simulink library "vco_snn"  (R2023b)
settings: Solver=VariableStepAuto  StartTime=0.0  StopTime=10.0  RelTol=1e-3
libraries: simulink_extras x166, spsSeriesRLCBranchLib x132, spsControlledVoltageSourceLib x126, $bdroot x33, fl_lib x18, msbPllFoundation x10, nesl_utility x9, spsVoltageMeasurementLib x8, simulink x6, spsGroundLib x5, eeGeneralControl x2
(part 2 of 2)

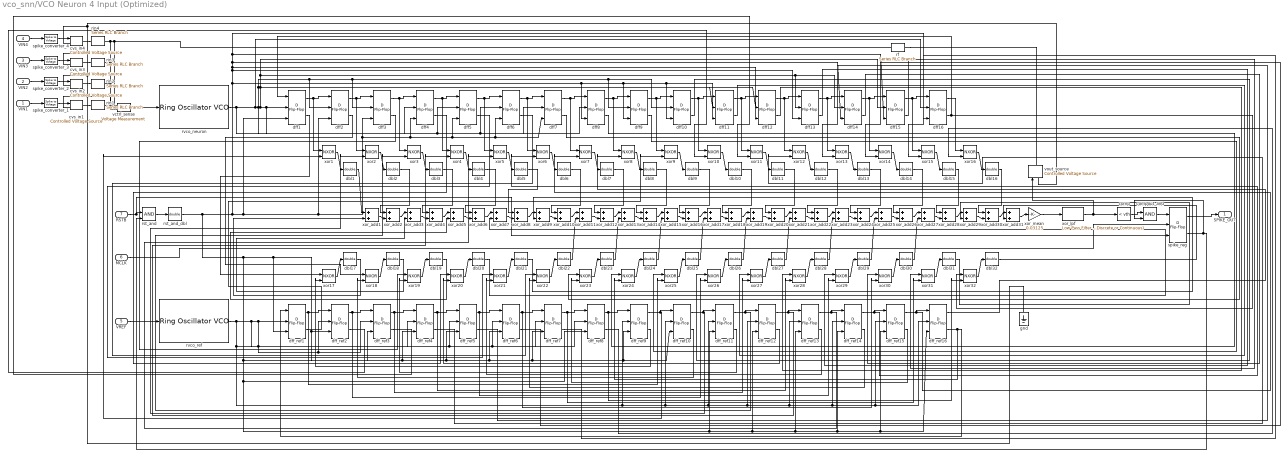
== system vco_snn/VCO Neuron 4 Input (Optimized) ==
  VIN1 : Inport
  VIN2 : Inport  Port=2
  VIN3 : Inport  Port=3
  VIN4 : Inport  Port=4
  VREF : Inport  Port=5
  MCLK : Inport  Port=6
  RSTB : Inport  Port=7
  comp : simulink/Logic and Bit Operations/Compare To Constant  relop=<  const=vth  OutDataTypeStr=boolean
  compout_and : Logic  IconShape=distinctive  AllPortsSameDT=off  OutDataTypeStr=boolean
  cvs_in{1..4} (4 alike) : spsControlledVoltageSourceLib/Controlled Voltage Source  Initialize=on  Source_Type=AC  Amplitude=0  Phase=0  Frequency=0  Measurements=None
  dbl{1..32} (32 alike) : DataTypeConversion  OutDataTypeStr=double  SaturateOnIntegerOverflow=off  RndMeth=Floor
  dff{1..16} (16 alike) : simulink_extras/Flip Flops/D Flip-Flop
  dff_ref{1..16} (16 alike) : simulink_extras/Flip Flops/D Flip-Flop
  gnd : spsGroundLib/Ground  LConnTagsString=a
  rf : spsSeriesRLCBranchLib/Series RLC Branch  LConnTagsString=__new0  RConnTagsString=__new0  BranchType=R  Resistance=rf  Inductance=1e-3  SetiL0=off  InitialCurrent=0  Capacitance=1e-6  Setx0=off  InitialVoltage=0  Measurements=None
  rin1 : spsSeriesRLCBranchLib/Series RLC Branch  LConnTagsString=__new0  RConnTagsString=__new0  BranchType=R  Resistance=rin1  Inductance=1e-3  SetiL0=off  InitialCurrent=0  Capacitance=1e-6  Setx0=off  InitialVoltage=0  Measurements=None
  rin2 : spsSeriesRLCBranchLib/Series RLC Branch  LConnTagsString=__new0  RConnTagsString=__new0  BranchType=R  Resistance=rin2  Inductance=1e-3  SetiL0=off  InitialCurrent=0  Capacitance=1e-6  Setx0=off  InitialVoltage=0  Measurements=None
  rin3 : spsSeriesRLCBranchLib/Series RLC Branch  LConnTagsString=__new0  RConnTagsString=__new0  BranchType=R  Resistance=rin3  Inductance=1e-3  SetiL0=off  InitialCurrent=0  Capacitance=1e-6  Setx0=off  InitialVoltage=0  Measurements=None
  rin4 : spsSeriesRLCBranchLib/Series RLC Branch  LConnTagsString=__new0  RConnTagsString=__new0  BranchType=R  Resistance=rin4  Inductance=1e-3  SetiL0=off  InitialCurrent=0  Capacitance=1e-6  Setx0=off  InitialVoltage=0  Measurements=None
  rst_and : Logic  IconShape=distinctive  AllPortsSameDT=off  OutDataTypeStr=boolean
  rst_and_dbl : DataTypeConversion  OutDataTypeStr=double  SaturateOnIntegerOverflow=off  RndMeth=Floor
  rvco_neuron : msbPllFoundation/Ring Oscillator VCO  SpecifyUsing=Voltage sensitivity  Kvco=kvco*32  Fo=(center_freq - (kvco/2))*32  ControlVoltage=[-5 0 5]  OutputFrequency=[2e9 2.5e9 3e9]  Amplitude=1  ExtraBuffer=off  NBuffer=10  AddPhaseNoise=off  SsbCheck=off  Foffset=[30e3 100e3 1e6 3e6 10e6]  PhaseNoise=[-56 -106 -132 -143 -152]  PeriodJitter=1.7e-15  CornerFrequency=5e5  CustomizeExponent=off  FlickerExponent=1.0  MaxKvco=320000000
  rvco_ref : msbPllFoundation/Ring Oscillator VCO  SpecifyUsing=Voltage sensitivity  Kvco=kvco*32  Fo=(center_freq - (kvco/2))*32  ControlVoltage=[-5 0 5]  OutputFrequency=[2e9 2.5e9 3e9]  Amplitude=1  ExtraBuffer=off  NBuffer=10  AddPhaseNoise=off  SsbCheck=off  Foffset=[30e3 100e3 1e6 3e6 10e6]  PhaseNoise=[-56 -106 -132 -143 -152]  PeriodJitter=1.7e-15  CornerFrequency=5e5  CustomizeExponent=off  FlickerExponent=1.0  MaxKvco=320000000
  spike_converter_1 : $bdroot/Spike to Voltage  vcm=vcm  spike_amp=spike_amp  sign=spike_sign1
  spike_converter_2 : $bdroot/Spike to Voltage  vcm=vcm  spike_amp=spike_amp  sign=spike_sign2
  spike_converter_3 : $bdroot/Spike to Voltage  vcm=vcm  spike_amp=spike_amp  sign=spike_sign3
  spike_converter_4 : $bdroot/Spike to Voltage  vcm=vcm  spike_amp=spike_amp  sign=spike_sign4
  spike_reg : simulink_extras/Flip Flops/D Flip-Flop
  vctrl_sense : spsVoltageMeasurementLib/Voltage Measurement  PhasorSimulation=off  OutputType=Complex  PSBequivalent=0
  vout_source : spsControlledVoltageSourceLib/Controlled Voltage Source  Initialize=on  Source_Type=AC  Amplitude=0  Phase=0  Frequency=0  Measurements=None
  xor{1..32} (32 alike) : Logic  Operator=NXOR  IconShape=distinctive  AllPortsSameDT=off  OutDataTypeStr=boolean
  xor_add{1..31} (31 alike) : Sum
  xor_lpf : eeGeneralControl/Low-Pass Filter (Discrete or Continuous)  K=1  T=xor_tau  B=inf  A=-inf  init_option=Inherited from block input  x0=0  Ts=0
  xor_mean : Gain  Gain=0.03125
  SPIKE_OUT : Outport
  wires:
  xor_add2/1 -> xor_add3/1
  dbl1/1 -> xor_add1/1
  xor17/1 -> dbl17/1
  dff_ref9/2 -> xor17/2
  spike_converter_2/1 -> cvs_in2/1
  xor8/1 -> dbl8/1
  dbl4/1 -> xor_add6/1
  xor_add5/1 -> xor_add6/2
  xor9/1 -> dbl9/1
  dff_ref13/2 -> xor21/2
  xor20/1 -> dbl20/1
  dff11/2 -> xor27/1
  dff10/2 -> xor26/1
  xor_add25/1 -> xor_add26/2
  dff4/2 -> xor20/1
  xor_add13/1 -> xor_add14/2
  dff_ref3/2 -> xor11/2
  spike_converter_3/1 -> cvs_in3/1
  dbl29/1 -> xor_add25/2
  xor18/1 -> dbl18/1
  xor_add4/1 -> xor_add5/1
  dbl9/1 -> xor_add16/1
  dff3/2 -> xor19/1
  dbl31/1 -> xor_add29/2
  dbl11/1 -> xor_add20/1
  spike_reg/2 -> compout_and/2, rst_and/2
  xor_add26/1 -> xor_add27/1
  dbl22/1 -> xor_add11/2
  xor_add15/1 -> xor_add16/2
  dff9/2 -> xor25/1
  dbl5/1 -> xor_add8/1
  xor7/1 -> dbl7/1
  xor3/1 -> dbl3/1
  xor5/1 -> dbl5/1
  xor_add7/1 -> xor_add8/2
  dff_ref11/2 -> xor19/2
  dff_ref8/2 -> xor16/2
  xor_add1/1 -> xor_add2/2
  spike_converter_4/1 -> cvs_in4/1
  dff_ref15/1 -> dff_ref16/1, xor7/2
  dff14/2 -> xor30/1
  xor_add12/1 -> xor_add13/1
  dbl23/1 -> xor_add13/2
  dff_ref5/2 -> xor13/2
  dbl13/1 -> xor_add24/1
  xor30/1 -> dbl30/1
  xor_add23/1 -> xor_add24/2
  xor22/1 -> dbl22/1
  xor12/1 -> dbl12/1
  xor15/1 -> dbl15/1
  dff_ref4/2 -> xor12/2
  dff_ref3/1 -> dff_ref4/1, xor27/2
  spike_reg/1 -> SPIKE_OUT/1
  xor24/1 -> dbl24/1
  xor_add9/1 -> xor_add10/2
  dff_ref12/1 -> dff_ref13/1, xor4/2
  xor28/1 -> dbl28/1
  xor_add19/1 -> xor_add20/2
  VIN1/1 -> spike_converter_1/1
  xor_add20/1 -> xor_add21/1
  xor_add11/1 -> xor_add12/2
  dff16/1 -> xor16/1
  dff6/1 -> dff7/1, xor6/1
  dff3/1 -> dff4/1, xor3/1
  dbl18/1 -> xor_add3/2
  xor27/1 -> dbl27/1
  xor_lpf/1 -> vout_source/1, comp/1
  dbl28/1 -> xor_add23/2
  dff_ref14/2 -> xor22/2
  dff1/1 -> dff2/1, xor1/1
  dbl3/1 -> xor_add4/1
  xor32/1 -> dbl32/1
  dff_ref15/2 -> xor23/2
  xor_add8/1 -> xor_add9/1
  xor_add6/1 -> xor_add7/1
  xor14/1 -> dbl14/1
  dff_ref11/1 -> dff_ref12/1, xor3/2
  xor1/1 -> dbl1/1
  dff6/2 -> xor22/1
  xor_add10/1 -> xor_add11/1
  dbl27/1 -> xor_add21/2
  xor16/1 -> dbl16/1
  xor29/1 -> dbl29/1
  dff15/1 -> dff16/1, xor15/1
  dff5/2 -> xor21/1
  dbl14/1 -> xor_add26/1
  xor_add21/1 -> xor_add22/2
  dbl17/1 -> xor_add1/2
  dff7/2 -> xor23/1
  dff_ref7/2 -> xor15/2
  dff14/1 -> dff15/1, xor14/1
  dff_ref16/1 -> xor8/2
  dff_ref1/1 -> dff_ref2/1, xor25/2
  dff_ref1/2 -> xor9/2
  rst_and/1 -> rst_and_dbl/1
  dbl19/1 -> xor_add5/2
  dbl6/1 -> xor_add10/1
  VIN2/1 -> spike_converter_2/1
  dff_ref9/1 -> dff_ref10/1, xor1/2
  dff_ref14/1 -> dff_ref15/1, xor6/2
  xor10/1 -> dbl10/1
  xor_mean/1 -> xor_lpf/1
  xor_add27/1 -> xor_add28/2
  dff_ref10/2 -> xor18/2
  xor2/1 -> dbl2/1
  dff16/2 -> dff1/1, xor32/1
  dbl20/1 -> xor_add7/2
  xor13/1 -> dbl13/1
  dbl16/1 -> xor_add30/1
  dff2/1 -> dff3/1, xor2/1
  dff10/1 -> dff11/1, xor10/1
  rst_and_dbl/1 -> dff_ref15/3, dff_ref16/3, dff_ref14/3, dff_ref13/3, dff_ref12/3, dff_ref11/3, dff_ref8/3, dff_ref9/3, dff_ref10/3, dff_ref7/3, dff_ref6/3, dff_ref5/3, dff_ref4/3, dff_ref2/3, dff_ref3/3, dff_ref1/3, dff6/3, dff7/3, dff5/3, dff4/3, dff3/3, dff2/3, dff1/3, dff10/3, dff11/3, dff9/3, dff8/3, dff15/3, dff16/3, dff14/3, dff12/3, dff13/3
  xor_add22/1 -> xor_add23/1
  dff_ref12/2 -> xor20/2
  RSTB/1 -> rst_and/1, spike_reg/3
  dff8/1 -> dff9/1, xor8/1
  dff_ref6/2 -> xor14/2
  xor_add31/1 -> xor_mean/1
  xor_add24/1 -> xor_add25/1
  xor_add30/1 -> xor_add31/1
  dbl25/1 -> xor_add17/2
  comp/1 -> compout_and/1
  dff_ref13/1 -> dff_ref14/1, xor5/2
  dff_ref8/1 -> dff_ref9/1, xor32/2
  xor_add29/1 -> xor_add30/2
  xor_add28/1 -> xor_add29/1
  dbl8/1 -> xor_add14/1
  dff_ref4/1 -> dff_ref5/1, xor28/2
  dff_ref10/1 -> dff_ref11/1, xor2/2
  VIN4/1 -> spike_converter_4/1
  xor31/1 -> dbl31/1
  dff11/1 -> dff12/1, xor11/1
  dff1/2 -> xor17/1
  xor11/1 -> dbl11/1
  dbl32/1 -> xor_add31/2
  dff12/1 -> dff13/1, xor12/1
  VIN3/1 -> spike_converter_3/1
  dff_ref16/2 -> dff_ref1/1, xor24/2
  dff7/1 -> dff8/1, xor7/1
  xor_add14/1 -> xor_add15/1
  spike_converter_1/1 -> cvs_in1/1
  dbl21/1 -> xor_add9/2
  dbl12/1 -> xor_add22/1
  xor25/1 -> dbl25/1
  dff4/1 -> dff5/1, xor4/1
  xor_add16/1 -> xor_add17/1
  xor_add17/1 -> xor_add18/2
  dff5/1 -> dff6/1, xor5/1
  dff8/2 -> xor24/1
  xor_add18/1 -> xor_add19/1
  rvco_neuron/1 -> dff6/2, dff7/2, dff5/2, dff1/2, dff8/2, dff13/2, dff14/2, dff15/2, dff12/2, dff9/2, dff10/2, dff3/2, dff2/2, dff11/2, dff4/2, dff16/2
  xor4/1 -> dbl4/1
  dff15/2 -> xor31/1
  xor19/1 -> dbl19/1
  dff13/2 -> xor29/1
  dff_ref6/1 -> dff_ref7/1, xor30/2
  dbl30/1 -> xor_add27/2
  dbl15/1 -> xor_add28/1
  dff_ref2/2 -> xor10/2
  dbl7/1 -> xor_add12/1
  dbl2/1 -> xor_add2/1
  dbl10/1 -> xor_add18/1
  dff13/1 -> dff14/1, xor13/1
  dff_ref2/1 -> dff_ref3/1, xor26/2
  dff12/2 -> xor28/1
  compout_and/1 -> spike_reg/1
  dff9/1 -> dff10/1, xor9/1
  xor_add3/1 -> xor_add4/2
  vctrl_sense/1 -> rvco_neuron/1
  dbl24/1 -> xor_add15/2
  rvco_ref/1 -> dff_ref15/2, dff_ref16/2, dff_ref14/2, dff_ref13/2, dff_ref12/2, dff_ref11/2, dff_ref10/2, dff_ref9/2, dff_ref8/2, dff_ref6/2, dff_ref7/2, dff_ref5/2, dff_ref2/2, dff_ref3/2, dff_ref4/2, dff_ref1/2
  dff_ref7/1 -> dff_ref8/1, xor31/2
  dff2/2 -> xor18/1
  dff_ref5/1 -> dff_ref6/1, xor29/2
  xor21/1 -> dbl21/1
  dbl26/1 -> xor_add19/2
  MCLK/1 -> spike_reg/2
  VREF/1 -> rvco_ref/1
  xor6/1 -> dbl6/1
  xor26/1 -> dbl26/1
  xor23/1 -> dbl23/1
  connections:
  cvs_in2/RConn1 -- rin2/LConn1
  rf/LConn1 -- rin1/RConn1 -- rin4/RConn1 -- rin3/RConn1 -- rin2/RConn1 -- vctrl_sense/LConn1
  cvs_in4/RConn1 -- rin4/LConn1
  rf/RConn1 -- vout_source/RConn1
  cvs_in3/RConn1 -- rin3/LConn1
  cvs_in1/RConn1 -- rin1/LConn1
  cvs_in1/LConn1 -- vctrl_sense/LConn2 -- gnd/LConn1 -- cvs_in2/LConn1 -- cvs_in3/LConn1 -- cvs_in4/LConn1 -- vout_source/LConn1

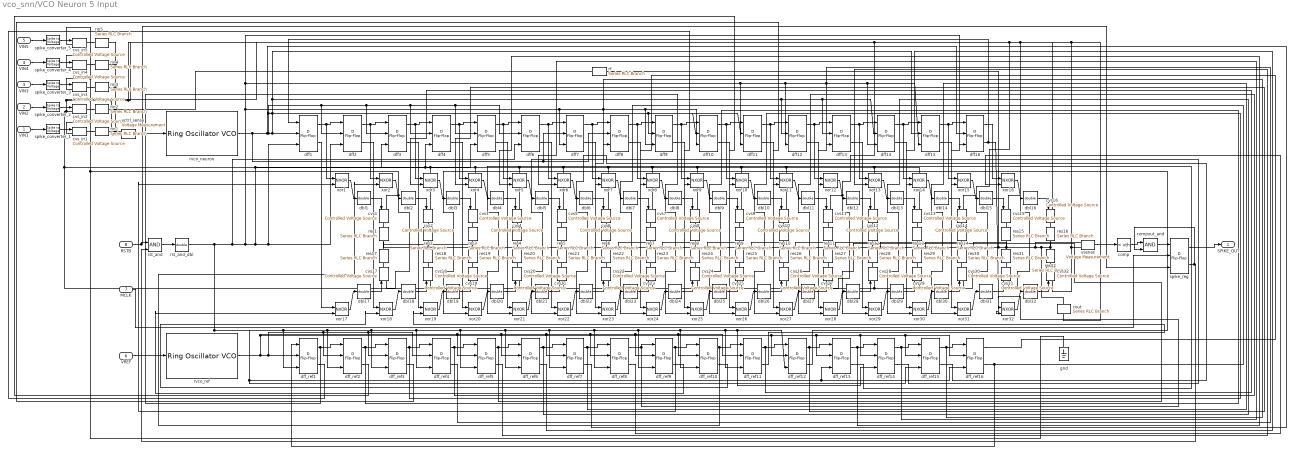
== system vco_snn/VCO Neuron 5 Input ==
  VIN1 : Inport
  VIN2 : Inport  Port=2
  VIN3 : Inport  Port=3
  VIN4 : Inport  Port=4
  VIN5 : Inport  Port=5
  VREF : Inport  Port=6
  MCLK : Inport  Port=7
  RSTB : Inport  Port=8
  comp : simulink/Logic and Bit Operations/Compare To Constant  relop=<  const=vth  OutDataTypeStr=boolean
  compout_and : Logic  IconShape=distinctive  AllPortsSameDT=off  OutDataTypeStr=boolean
  cout : spsSeriesRLCBranchLib/Series RLC Branch  LConnTagsString=__new0  RConnTagsString=__new0  BranchType=C  Resistance=1  Inductance=1e-3  SetiL0=off  InitialCurrent=0  Capacitance=vout_cap  Setx0=on  InitialVoltage=0.5  Measurements=None
  cvs{1..32} (32 alike) : spsControlledVoltageSourceLib/Controlled Voltage Source  Initialize=on  Source_Type=AC  Amplitude=0  Phase=0  Frequency=0  Measurements=None
  cvs_in{1..5} (5 alike) : spsControlledVoltageSourceLib/Controlled Voltage Source  Initialize=on  Source_Type=AC  Amplitude=0  Phase=0  Frequency=0  Measurements=None
  dbl{1..32} (32 alike) : DataTypeConversion  OutDataTypeStr=double  SaturateOnIntegerOverflow=off  RndMeth=Floor
  dff{1..16} (16 alike) : simulink_extras/Flip Flops/D Flip-Flop
  dff_ref{1..16} (16 alike) : simulink_extras/Flip Flops/D Flip-Flop
  gnd : spsGroundLib/Ground  LConnTagsString=a
  res{1..32} (32 alike) : spsSeriesRLCBranchLib/Series RLC Branch  LConnTagsString=__new0  RConnTagsString=__new0  BranchType=R  Resistance=xor_res  Inductance=1e-3  SetiL0=off  InitialCurrent=0  Capacitance=1e-6  Setx0=off  InitialVoltage=0  Measurements=None
  rf : spsSeriesRLCBranchLib/Series RLC Branch  LConnTagsString=__new0  RConnTagsString=__new0  BranchType=R  Resistance=rf  Inductance=1e-3  SetiL0=off  InitialCurrent=0  Capacitance=1e-6  Setx0=off  InitialVoltage=0  Measurements=None
  rin1 : spsSeriesRLCBranchLib/Series RLC Branch  LConnTagsString=__new0  RConnTagsString=__new0  BranchType=R  Resistance=rin1  Inductance=1e-3  SetiL0=off  InitialCurrent=0  Capacitance=1e-6  Setx0=off  InitialVoltage=0  Measurements=None
  rin2 : spsSeriesRLCBranchLib/Series RLC Branch  LConnTagsString=__new0  RConnTagsString=__new0  BranchType=R  Resistance=rin2  Inductance=1e-3  SetiL0=off  InitialCurrent=0  Capacitance=1e-6  Setx0=off  InitialVoltage=0  Measurements=None
  rin3 : spsSeriesRLCBranchLib/Series RLC Branch  LConnTagsString=__new0  RConnTagsString=__new0  BranchType=R  Resistance=rin3  Inductance=1e-3  SetiL0=off  InitialCurrent=0  Capacitance=1e-6  Setx0=off  InitialVoltage=0  Measurements=None
  rin4 : spsSeriesRLCBranchLib/Series RLC Branch  LConnTagsString=__new0  RConnTagsString=__new0  BranchType=R  Resistance=rin4  Inductance=1e-3  SetiL0=off  InitialCurrent=0  Capacitance=1e-6  Setx0=off  InitialVoltage=0  Measurements=None
  rin5 : spsSeriesRLCBranchLib/Series RLC Branch  LConnTagsString=__new0  RConnTagsString=__new0  BranchType=R  Resistance=rin5  Inductance=1e-3  SetiL0=off  InitialCurrent=0  Capacitance=1e-6  Setx0=off  InitialVoltage=0  Measurements=None
  rst_and : Logic  IconShape=distinctive  AllPortsSameDT=off  OutDataTypeStr=boolean
  rst_and_dbl : DataTypeConversion  OutDataTypeStr=double  SaturateOnIntegerOverflow=off  RndMeth=Floor
  rvco_neuron : msbPllFoundation/Ring Oscillator VCO  SpecifyUsing=Voltage sensitivity  Kvco=kvco*32  Fo=(center_freq - (kvco/2))*32  ControlVoltage=[-5 0 5]  OutputFrequency=[2e9 2.5e9 3e9]  Amplitude=1  ExtraBuffer=off  NBuffer=10  AddPhaseNoise=off  SsbCheck=off  Foffset=[30e3 100e3 1e6 3e6 10e6]  PhaseNoise=[-56 -106 -132 -143 -152]  PeriodJitter=1.7e-15  CornerFrequency=5e5  CustomizeExponent=off  FlickerExponent=1.0  MaxKvco=320000000
  rvco_ref : msbPllFoundation/Ring Oscillator VCO  SpecifyUsing=Voltage sensitivity  Kvco=kvco*32  Fo=(center_freq - (kvco/2))*32  ControlVoltage=[-5 0 5]  OutputFrequency=[2e9 2.5e9 3e9]  Amplitude=1  ExtraBuffer=off  NBuffer=10  AddPhaseNoise=off  SsbCheck=off  Foffset=[30e3 100e3 1e6 3e6 10e6]  PhaseNoise=[-56 -106 -132 -143 -152]  PeriodJitter=1.7e-15  CornerFrequency=5e5  CustomizeExponent=off  FlickerExponent=1.0  MaxKvco=320000000
  spike_converter_1 : $bdroot/Spike to Voltage  vcm=vcm  spike_amp=spike_amp  sign=spike_sign1
  spike_converter_2 : $bdroot/Spike to Voltage  vcm=vcm  spike_amp=spike_amp  sign=spike_sign2
  spike_converter_3 : $bdroot/Spike to Voltage  vcm=vcm  spike_amp=spike_amp  sign=spike_sign3
  spike_converter_4 : $bdroot/Spike to Voltage  vcm=vcm  spike_amp=spike_amp  sign=spike_sign4
  spike_converter_5 : $bdroot/Spike to Voltage  vcm=vcm  spike_amp=spike_amp  sign=spike_sign5
  spike_reg : simulink_extras/Flip Flops/D Flip-Flop
  vctrl_sense : spsVoltageMeasurementLib/Voltage Measurement  PhasorSimulation=off  OutputType=Complex  PSBequivalent=0
  vsense : spsVoltageMeasurementLib/Voltage Measurement  PhasorSimulation=off  OutputType=Complex  PSBequivalent=0
  xor{1..32} (32 alike) : Logic  Operator=NXOR  IconShape=distinctive  AllPortsSameDT=off  OutDataTypeStr=boolean
  SPIKE_OUT : Outport
  wires:
  xor31/1 -> dbl31/1
  dbl17/1 -> cvs17/1
  xor8/1 -> dbl8/1
  xor18/1 -> dbl18/1
  dbl19/1 -> cvs19/1
  xor17/1 -> dbl17/1
  xor22/1 -> dbl22/1
  dbl21/1 -> cvs21/1
  dbl6/1 -> cvs6/1
  dff_ref15/2 -> xor23/2
  dbl7/1 -> cvs7/1
  dbl5/1 -> cvs5/1
  xor30/1 -> dbl30/1
  xor3/1 -> dbl3/1
  VREF/1 -> rvco_ref/1
  dff11/2 -> xor27/1
  dff2/1 -> dff3/1, xor2/1
  xor25/1 -> dbl25/1
  xor24/1 -> dbl24/1
  spike_reg/1 -> SPIKE_OUT/1
  dff_ref16/2 -> dff_ref1/1, xor24/2
  rst_and/1 -> rst_and_dbl/1
  dbl3/1 -> cvs3/1
  dff8/1 -> dff9/1, xor8/1
  dff_ref9/2 -> xor17/2
  dff4/2 -> xor20/1
  dbl15/1 -> cvs15/1
  dff8/2 -> xor24/1
  xor32/1 -> dbl32/1
  dbl18/1 -> cvs18/1
  dff_ref13/1 -> dff_ref14/1, xor5/2
  dff3/2 -> xor19/1
  dbl10/1 -> cvs10/1
  dbl26/1 -> cvs26/1
  dff_ref7/2 -> xor15/2
  dbl25/1 -> cvs25/1
  dbl24/1 -> cvs24/1
  xor12/1 -> dbl12/1
  xor28/1 -> dbl28/1
  VIN5/1 -> spike_converter_5/1
  dff12/2 -> xor28/1
  dbl22/1 -> cvs22/1
  compout_and/1 -> spike_reg/1
  dbl13/1 -> cvs13/1
  dff_ref7/1 -> dff_ref8/1, xor31/2
  dff3/1 -> dff4/1, xor3/1
  dff_ref15/1 -> dff_ref16/1, xor7/2
  xor19/1 -> dbl19/1
  dff14/2 -> xor30/1
  xor15/1 -> dbl15/1
  spike_converter_3/1 -> cvs_in3/1
  dff_ref9/1 -> dff_ref10/1, xor1/2
  dbl16/1 -> cvs16/1
  dff_ref3/1 -> dff_ref4/1, xor27/2
  dff13/1 -> dff14/1, xor13/1
  dff9/1 -> dff10/1, xor9/1
  xor14/1 -> dbl14/1
  dff1/1 -> dff2/1, xor1/1
  dff_ref2/1 -> dff_ref3/1, xor26/2
  dff5/1 -> dff6/1, xor5/1
  dff_ref5/1 -> dff_ref6/1, xor29/2
  dff_ref11/1 -> dff_ref12/1, xor3/2
  spike_reg/2 -> compout_and/2, rst_and/2
  dff6/1 -> dff7/1, xor6/1
  dff12/1 -> dff13/1, xor12/1
  dff_ref8/2 -> xor16/2
  spike_converter_5/1 -> cvs_in5/1
  dbl1/1 -> cvs1/1
  dff16/1 -> xor16/1
  dff_ref12/1 -> dff_ref13/1, xor4/2
  dff10/1 -> dff11/1, xor10/1
  dff10/2 -> xor26/1
  dff_ref1/1 -> dff_ref2/1, xor25/2
  xor20/1 -> dbl20/1
  dff14/1 -> dff15/1, xor14/1
  VIN3/1 -> spike_converter_3/1
  dff13/2 -> xor29/1
  dff_ref14/2 -> xor22/2
  dff_ref3/2 -> xor11/2
  spike_converter_2/1 -> cvs_in2/1
  VIN4/1 -> spike_converter_4/1
  xor27/1 -> dbl27/1
  vsense/1 -> comp/1
  spike_converter_4/1 -> cvs_in4/1
  RSTB/1 -> rst_and/1, spike_reg/3
  dff7/1 -> dff8/1, xor7/1
  xor7/1 -> dbl7/1
  dff_ref6/1 -> dff_ref7/1, xor30/2
  dff_ref14/1 -> dff_ref15/1, xor6/2
  comp/1 -> compout_and/1
  xor9/1 -> dbl9/1
  dff16/2 -> dff1/1, xor32/1
  dff_ref4/1 -> dff_ref5/1, xor28/2
  xor5/1 -> dbl5/1
  dbl32/1 -> cvs32/1
  xor13/1 -> dbl13/1
  dff_ref5/2 -> xor13/2
  xor11/1 -> dbl11/1
  dbl2/1 -> cvs2/1
  xor16/1 -> dbl16/1
  xor2/1 -> dbl2/1
  xor21/1 -> dbl21/1
  dff15/2 -> xor31/1
  vctrl_sense/1 -> rvco_neuron/1
  dbl8/1 -> cvs8/1
  dff1/2 -> xor17/1
  xor4/1 -> dbl4/1
  VIN1/1 -> spike_converter_1/1
  dff_ref1/2 -> xor9/2
  MCLK/1 -> spike_reg/2
  dff5/2 -> xor21/1
  dbl29/1 -> cvs29/1
  xor29/1 -> dbl29/1
  dff_ref12/2 -> xor20/2
  dff15/1 -> dff16/1, xor15/1
  dbl30/1 -> cvs30/1
  dff_ref11/2 -> xor19/2
  dbl9/1 -> cvs9/1
  xor6/1 -> dbl6/1
  spike_converter_1/1 -> cvs_in1/1
  dbl28/1 -> cvs28/1
  rst_and_dbl/1 -> dff_ref13/3, dff_ref16/3, dff_ref15/3, dff_ref12/3, dff_ref14/3, dff_ref11/3, dff_ref10/3, dff_ref9/3, dff_ref8/3, dff_ref7/3, dff_ref6/3, dff_ref5/3, dff_ref4/3, dff_ref3/3, dff_ref2/3, dff_ref1/3, dff1/3, dff2/3, dff4/3, dff5/3, dff3/3, dff9/3, dff10/3, dff8/3, dff7/3, dff14/3, dff15/3, dff13/3, dff12/3, dff11/3, dff16/3, dff6/3
  dff7/2 -> xor23/1
  xor10/1 -> dbl10/1
  rvco_ref/1 -> dff_ref3/2, dff_ref4/2, dff_ref2/2, dff_ref1/2, dff_ref15/2, dff_ref16/2, dff_ref14/2, dff_ref13/2, dff_ref12/2, dff_ref10/2, dff_ref11/2, dff_ref9/2, dff_ref8/2, dff_ref7/2, dff_ref6/2, dff_ref5/2
  VIN2/1 -> spike_converter_2/1
  xor26/1 -> dbl26/1
  dbl4/1 -> cvs4/1
  dff_ref2/2 -> xor10/2
  dff_ref16/1 -> xor8/2
  dbl11/1 -> cvs11/1
  dff_ref8/1 -> dff_ref9/1, xor32/2
  xor1/1 -> dbl1/1
  dbl31/1 -> cvs31/1
  dff_ref13/2 -> xor21/2
  dff6/2 -> xor22/1
  xor23/1 -> dbl23/1
  dbl20/1 -> cvs20/1
  dbl12/1 -> cvs12/1
  dbl23/1 -> cvs23/1
  dff11/1 -> dff12/1, xor11/1
  dff9/2 -> xor25/1
  dff_ref4/2 -> xor12/2
  dff_ref6/2 -> xor14/2
  dff4/1 -> dff5/1, xor4/1
  dbl14/1 -> cvs14/1
  rvco_neuron/1 -> dff7/2, dff8/2, dff13/2, dff14/2, dff12/2, dff15/2, dff11/2, dff1/2, dff9/2, dff10/2, dff5/2, dff6/2, dff4/2, dff3/2, dff2/2, dff16/2
  dff_ref10/2 -> xor18/2
  dbl27/1 -> cvs27/1
  dff2/2 -> xor18/1
  dff_ref10/1 -> dff_ref11/1, xor2/2
  connections:
  cvs21/RConn1 -- res21/RConn1
  cvs27/RConn1 -- res27/RConn1
  cvs18/RConn1 -- res18/RConn1
  cvs30/RConn1 -- res30/RConn1
  cvs2/RConn1 -- res2/RConn1
  cvs25/RConn1 -- res25/RConn1
  cvs15/RConn1 -- res15/RConn1
  cvs23/RConn1 -- res23/RConn1
  cvs8/RConn1 -- res8/RConn1
  cvs5/RConn1 -- res5/RConn1
  cvs16/RConn1 -- res16/RConn1
  cvs28/RConn1 -- res28/RConn1
  cvs_in4/RConn1 -- rin4/LConn1
  cvs14/RConn1 -- res14/RConn1
  cvs10/RConn1 -- res10/RConn1
  cvs31/RConn1 -- res31/RConn1
  cvs11/RConn1 -- res11/RConn1
  cvs_in1/RConn1 -- rin1/LConn1
  cvs3/RConn1 -- res3/RConn1
  cvs4/RConn1 -- res4/RConn1
  cvs9/RConn1 -- res9/RConn1
  rin1/RConn1 -- vctrl_sense/LConn1 -- rin2/RConn1 -- rf/LConn1 -- rin3/RConn1 -- rin5/RConn1 -- rin4/RConn1
  cvs7/RConn1 -- res7/RConn1
  cvs12/RConn1 -- res12/RConn1
  cvs32/RConn1 -- res32/RConn1
  cvs19/RConn1 -- res19/RConn1
  cvs26/RConn1 -- res26/RConn1
  cvs_in2/RConn1 -- rin2/LConn1
  cvs20/RConn1 -- res20/RConn1
  cvs13/RConn1 -- res13/RConn1
  cvs29/RConn1 -- res29/RConn1
  cvs24/RConn1 -- res24/RConn1
  cvs13/LConn1 -- cvs12/LConn1 -- cvs10/LConn1 -- cvs9/LConn1 -- cvs8/LConn1 -- cvs7/LConn1 -- cvs6/LConn1 -- cvs5/LConn1 -- cvs4/LConn1 -- cvs3/LConn1 -- cvs2/LConn1 -- cvs17/LConn1 -- cvs1/LConn1 -- gnd/LConn1 -- cvs_in1/LConn1 -- cvs27/LConn1 -- cvs11/LConn1 -- cvs15/LConn1 -- cvs14/LConn1 -- cvs32/LConn1 -- vsense/LConn2 -- cout/RConn1 -- cvs31/LConn1 -- cvs30/LConn1 -- vctrl_sense/LConn2 -- cvs_in5/LConn1 -- cvs_in4/LConn1 -- cvs_in3/LConn1 -- cvs16/LConn1 -- cvs_in2/LConn1 -- cvs18/LConn1 -- cvs19/LConn1 -- cvs20/LConn1 -- cvs21/LConn1 -- cvs22/LConn1 -- cvs23/LConn1 -- cvs24/LConn1 -- cvs25/LConn1 -- cvs26/LConn1 -- cvs29/LConn1 -- cvs28/LConn1
  cvs_in3/RConn1 -- rin3/LConn1
  cvs_in5/RConn1 -- rin5/LConn1
  cvs22/RConn1 -- res22/RConn1
  cvs17/RConn1 -- res17/RConn1
  cvs1/RConn1 -- res1/RConn1
  res2/LConn1 -- res1/LConn1 -- res18/LConn1 -- res17/LConn1 -- res19/LConn1 -- res3/LConn1 -- res20/LConn1 -- res4/LConn1 -- res21/LConn1 -- res5/LConn1 -- res22/LConn1 -- res6/LConn1 -- res23/LConn1 -- res7/LConn1 -- res24/LConn1 -- res8/LConn1 -- res25/LConn1 -- res9/LConn1 -- res26/LConn1 -- res10/LConn1 -- res27/LConn1 -- res11/LConn1 -- res28/LConn1 -- res12/LConn1 -- res29/LConn1 -- res13/LConn1 -- res30/LConn1 -- res14/LConn1 -- res31/LConn1 -- rf/RConn1 -- res15/LConn1 -- vsense/LConn1 -- cout/LConn1 -- res32/LConn1 -- res16/LConn1
  cvs6/RConn1 -- res6/RConn1

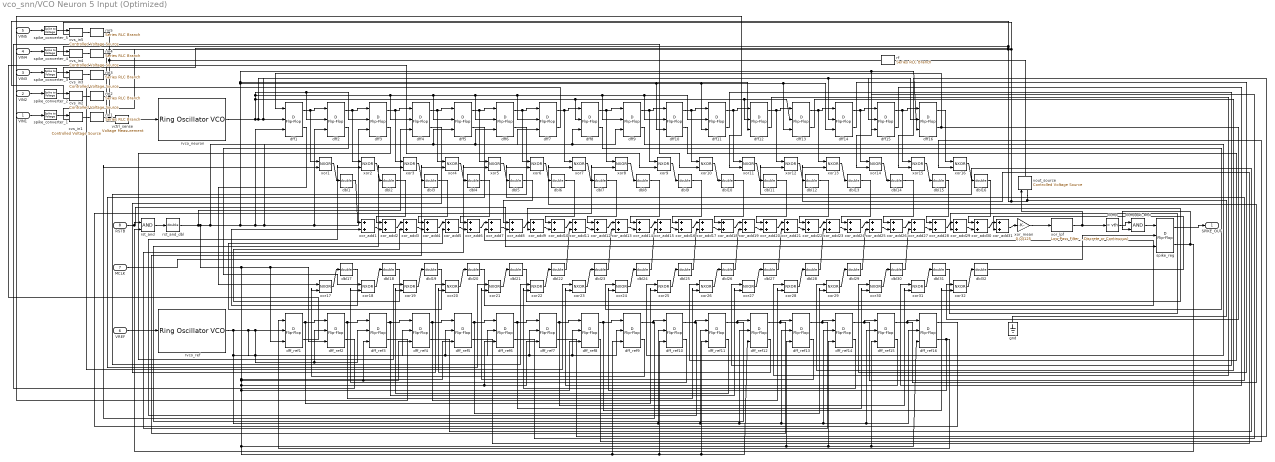
== system vco_snn/VCO Neuron 5 Input (Optimized) ==
  VIN1 : Inport
  VIN2 : Inport  Port=2
  VIN3 : Inport  Port=3
  VIN4 : Inport  Port=4
  VIN5 : Inport  Port=5
  VREF : Inport  Port=6
  MCLK : Inport  Port=7
  RSTB : Inport  Port=8
  comp : simulink/Logic and Bit Operations/Compare To Constant  relop=<  const=vth  OutDataTypeStr=boolean
  compout_and : Logic  IconShape=distinctive  AllPortsSameDT=off  OutDataTypeStr=boolean
  cvs_in{1..5} (5 alike) : spsControlledVoltageSourceLib/Controlled Voltage Source  Initialize=on  Source_Type=AC  Amplitude=0  Phase=0  Frequency=0  Measurements=None
  dbl{1..32} (32 alike) : DataTypeConversion  OutDataTypeStr=double  SaturateOnIntegerOverflow=off  RndMeth=Floor
  dff{1..16} (16 alike) : simulink_extras/Flip Flops/D Flip-Flop
  dff_ref{1..16} (16 alike) : simulink_extras/Flip Flops/D Flip-Flop
  gnd : spsGroundLib/Ground  LConnTagsString=a
  rf : spsSeriesRLCBranchLib/Series RLC Branch  LConnTagsString=__new0  RConnTagsString=__new0  BranchType=R  Resistance=rf  Inductance=1e-3  SetiL0=off  InitialCurrent=0  Capacitance=1e-6  Setx0=off  InitialVoltage=0  Measurements=None
  rin1 : spsSeriesRLCBranchLib/Series RLC Branch  LConnTagsString=__new0  RConnTagsString=__new0  BranchType=R  Resistance=rin1  Inductance=1e-3  SetiL0=off  InitialCurrent=0  Capacitance=1e-6  Setx0=off  InitialVoltage=0  Measurements=None
  rin2 : spsSeriesRLCBranchLib/Series RLC Branch  LConnTagsString=__new0  RConnTagsString=__new0  BranchType=R  Resistance=rin2  Inductance=1e-3  SetiL0=off  InitialCurrent=0  Capacitance=1e-6  Setx0=off  InitialVoltage=0  Measurements=None
  rin3 : spsSeriesRLCBranchLib/Series RLC Branch  LConnTagsString=__new0  RConnTagsString=__new0  BranchType=R  Resistance=rin3  Inductance=1e-3  SetiL0=off  InitialCurrent=0  Capacitance=1e-6  Setx0=off  InitialVoltage=0  Measurements=None
  rin4 : spsSeriesRLCBranchLib/Series RLC Branch  LConnTagsString=__new0  RConnTagsString=__new0  BranchType=R  Resistance=rin4  Inductance=1e-3  SetiL0=off  InitialCurrent=0  Capacitance=1e-6  Setx0=off  InitialVoltage=0  Measurements=None
  rin5 : spsSeriesRLCBranchLib/Series RLC Branch  LConnTagsString=__new0  RConnTagsString=__new0  BranchType=R  Resistance=rin5  Inductance=1e-3  SetiL0=off  InitialCurrent=0  Capacitance=1e-6  Setx0=off  InitialVoltage=0  Measurements=None
  rst_and : Logic  IconShape=distinctive  AllPortsSameDT=off  OutDataTypeStr=boolean
  rst_and_dbl : DataTypeConversion  OutDataTypeStr=double  SaturateOnIntegerOverflow=off  RndMeth=Floor
  rvco_neuron : msbPllFoundation/Ring Oscillator VCO  SpecifyUsing=Voltage sensitivity  Kvco=kvco*32  Fo=(center_freq - (kvco/2))*32  ControlVoltage=[-5 0 5]  OutputFrequency=[2e9 2.5e9 3e9]  Amplitude=1  ExtraBuffer=off  NBuffer=10  AddPhaseNoise=off  SsbCheck=off  Foffset=[30e3 100e3 1e6 3e6 10e6]  PhaseNoise=[-56 -106 -132 -143 -152]  PeriodJitter=1.7e-15  CornerFrequency=5e5  CustomizeExponent=off  FlickerExponent=1.0  MaxKvco=320000000
  rvco_ref : msbPllFoundation/Ring Oscillator VCO  SpecifyUsing=Voltage sensitivity  Kvco=kvco*32  Fo=(center_freq - (kvco/2))*32  ControlVoltage=[-5 0 5]  OutputFrequency=[2e9 2.5e9 3e9]  Amplitude=1  ExtraBuffer=off  NBuffer=10  AddPhaseNoise=off  SsbCheck=off  Foffset=[30e3 100e3 1e6 3e6 10e6]  PhaseNoise=[-56 -106 -132 -143 -152]  PeriodJitter=1.7e-15  CornerFrequency=5e5  CustomizeExponent=off  FlickerExponent=1.0  MaxKvco=320000000
  spike_converter_1 : $bdroot/Spike to Voltage  vcm=vcm  spike_amp=spike_amp  sign=spike_sign1
  spike_converter_2 : $bdroot/Spike to Voltage  vcm=vcm  spike_amp=spike_amp  sign=spike_sign2
  spike_converter_3 : $bdroot/Spike to Voltage  vcm=vcm  spike_amp=spike_amp  sign=spike_sign3
  spike_converter_4 : $bdroot/Spike to Voltage  vcm=vcm  spike_amp=spike_amp  sign=spike_sign4
  spike_converter_5 : $bdroot/Spike to Voltage  vcm=vcm  spike_amp=spike_amp  sign=spike_sign5
  spike_reg : simulink_extras/Flip Flops/D Flip-Flop
  vctrl_sense : spsVoltageMeasurementLib/Voltage Measurement  PhasorSimulation=off  OutputType=Complex  PSBequivalent=0
  vout_source : spsControlledVoltageSourceLib/Controlled Voltage Source  Initialize=on  Source_Type=AC  Amplitude=0  Phase=0  Frequency=0  Measurements=None
  xor{1..32} (32 alike) : Logic  Operator=NXOR  IconShape=distinctive  AllPortsSameDT=off  OutDataTypeStr=boolean
  xor_add{1..31} (31 alike) : Sum
  xor_lpf : eeGeneralControl/Low-Pass Filter (Discrete or Continuous)  K=1  T=xor_tau  B=inf  A=-inf  init_option=Inherited from block input  x0=0  Ts=0
  xor_mean : Gain  Gain=0.03125
  SPIKE_OUT : Outport
  wires:
  xor_add27/1 -> xor_add28/2
  dbl12/1 -> xor_add22/1
  dbl25/1 -> xor_add17/2
  xor_add15/1 -> xor_add16/2
  xor_add10/1 -> xor_add11/1
  xor_add30/1 -> xor_add31/1
  xor_add24/1 -> xor_add25/1
  dbl13/1 -> xor_add24/1
  dff14/2 -> xor30/1
  dff16/1 -> xor16/1
  dbl5/1 -> xor_add8/1
  xor10/1 -> dbl10/1
  xor3/1 -> dbl3/1
  xor_add1/1 -> xor_add2/2
  xor_add26/1 -> xor_add27/1
  xor31/1 -> dbl31/1
  dbl20/1 -> xor_add7/2
  dbl17/1 -> xor_add1/2
  xor_add2/1 -> xor_add3/1
  dff13/2 -> xor29/1
  xor_mean/1 -> xor_lpf/1
  xor30/1 -> dbl30/1
  dff_ref6/2 -> xor14/2
  dbl2/1 -> xor_add2/1
  xor_add31/1 -> xor_mean/1
  xor32/1 -> dbl32/1
  compout_and/1 -> spike_reg/1
  xor16/1 -> dbl16/1
  xor23/1 -> dbl23/1
  xor4/1 -> dbl4/1
  VIN2/1 -> spike_converter_2/1
  dbl31/1 -> xor_add29/2
  dff_ref2/1 -> dff_ref3/1, xor26/2
  xor_add7/1 -> xor_add8/2
  xor_add9/1 -> xor_add10/2
  dff12/2 -> xor28/1
  xor_add6/1 -> xor_add7/1
  dff_ref7/1 -> dff_ref8/1, xor31/2
  dff15/1 -> dff16/1, xor15/1
  dbl11/1 -> xor_add20/1
  dbl22/1 -> xor_add11/2
  xor_add28/1 -> xor_add29/1
  xor15/1 -> dbl15/1
  dff_ref9/1 -> dff_ref10/1, xor1/2
  dff9/1 -> dff10/1, xor9/1
  dff15/2 -> xor31/1
  dff_ref11/2 -> xor19/2
  dbl21/1 -> xor_add9/2
  dff_ref5/2 -> xor13/2
  dbl7/1 -> xor_add12/1
  xor_add19/1 -> xor_add20/2
  xor17/1 -> dbl17/1
  VIN4/1 -> spike_converter_4/1
  xor21/1 -> dbl21/1
  dff2/1 -> dff3/1, xor2/1
  dbl23/1 -> xor_add13/2
  xor_add29/1 -> xor_add30/2
  VIN3/1 -> spike_converter_3/1
  xor_add8/1 -> xor_add9/1
  xor8/1 -> dbl8/1
  xor1/1 -> dbl1/1
  xor25/1 -> dbl25/1
  VIN1/1 -> spike_converter_1/1
  dbl4/1 -> xor_add6/1
  xor7/1 -> dbl7/1
  xor9/1 -> dbl9/1
  dff_ref14/2 -> xor22/2
  xor6/1 -> dbl6/1
  dbl30/1 -> xor_add27/2
  dff_ref15/1 -> dff_ref16/1, xor7/2
  xor22/1 -> dbl22/1
  dff_ref1/1 -> dff_ref2/1, xor25/2
  dff5/2 -> xor21/1
  dbl14/1 -> xor_add26/1
  xor_add5/1 -> xor_add6/2
  dff_ref1/2 -> xor9/2
  xor_add13/1 -> xor_add14/2
  dff14/1 -> dff15/1, xor14/1
  dff_ref16/1 -> xor8/2
  dff8/1 -> dff9/1, xor8/1
  dff_ref4/2 -> xor12/2
  dff_ref10/2 -> xor18/2
  spike_converter_2/1 -> cvs_in2/1
  vctrl_sense/1 -> rvco_neuron/1
  dff10/2 -> xor26/1
  xor26/1 -> dbl26/1
  dff6/1 -> dff7/1, xor6/1
  dbl28/1 -> xor_add23/2
  xor24/1 -> dbl24/1
  xor12/1 -> dbl12/1
  dbl8/1 -> xor_add14/1
  VREF/1 -> rvco_ref/1
  xor_add3/1 -> xor_add4/2
  dbl26/1 -> xor_add19/2
  dbl18/1 -> xor_add3/2
  dff_ref6/1 -> dff_ref7/1, xor30/2
  dff_ref7/2 -> xor15/2
  MCLK/1 -> spike_reg/2
  dff11/2 -> xor27/1
  dff3/1 -> dff4/1, xor3/1
  dbl27/1 -> xor_add21/2
  dff_ref12/2 -> xor20/2
  dff7/2 -> xor23/1
  xor_add4/1 -> xor_add5/1
  dbl15/1 -> xor_add28/1
  dbl1/1 -> xor_add1/1
  dbl10/1 -> xor_add18/1
  dff1/1 -> dff2/1, xor1/1
  xor13/1 -> dbl13/1
  xor_add17/1 -> xor_add18/2
  xor_add20/1 -> xor_add21/1
  comp/1 -> compout_and/1
  xor_add12/1 -> xor_add13/1
  dff_ref3/1 -> dff_ref4/1, xor27/2
  dff8/2 -> xor24/1
  xor2/1 -> dbl2/1
  dff4/1 -> dff5/1, xor4/1
  dff9/2 -> xor25/1
  spike_reg/2 -> compout_and/2, rst_and/2
  dff1/2 -> xor17/1
  xor5/1 -> dbl5/1
  xor_add14/1 -> xor_add15/1
  dff3/2 -> xor19/1
  dff_ref11/1 -> dff_ref12/1, xor3/2
  rvco_neuron/1 -> dff14/2, dff15/2, dff1/2, dff16/2, dff12/2, dff13/2, dff8/2, dff10/2, dff11/2, dff9/2, dff7/2, dff6/2, dff5/2, dff4/2, dff2/2, dff3/2
  dff_ref2/2 -> xor10/2
  xor_add25/1 -> xor_add26/2
  xor_add22/1 -> xor_add23/1
  dbl32/1 -> xor_add31/2
  VIN5/1 -> spike_converter_5/1
  dff_ref15/2 -> xor23/2
  dff_ref14/1 -> dff_ref15/1, xor6/2
  dff6/2 -> xor22/1
  dff13/1 -> dff14/1, xor13/1
  RSTB/1 -> rst_and/1, spike_reg/3
  spike_converter_3/1 -> cvs_in3/1
  xor_lpf/1 -> vout_source/1, comp/1
  xor18/1 -> dbl18/1
  dbl16/1 -> xor_add30/1
  dff11/1 -> dff12/1, xor11/1
  dff5/1 -> dff6/1, xor5/1
  dff_ref13/1 -> dff_ref14/1, xor5/2
  rvco_ref/1 -> dff_ref15/2, dff_ref16/2, dff_ref14/2, dff_ref13/2, dff_ref12/2, dff_ref11/2, dff_ref10/2, dff_ref8/2, dff_ref9/2, dff_ref7/2, dff_ref5/2, dff_ref6/2, dff_ref2/2, dff_ref3/2, dff_ref4/2, dff_ref1/2
  xor_add16/1 -> xor_add17/1
  xor11/1 -> dbl11/1
  xor19/1 -> dbl19/1
  dbl19/1 -> xor_add5/2
  dff_ref4/1 -> dff_ref5/1, xor28/2
  dff_ref10/1 -> dff_ref11/1, xor2/2
  xor27/1 -> dbl27/1
  dbl29/1 -> xor_add25/2
  dff12/1 -> dff13/1, xor12/1
  rst_and/1 -> rst_and_dbl/1
  xor_add18/1 -> xor_add19/1
  rst_and_dbl/1 -> dff_ref11/3, dff_ref12/3, dff_ref10/3, dff_ref9/3, dff_ref15/3, dff_ref16/3, dff_ref14/3, dff_ref13/3, dff_ref8/3, dff_ref6/3, dff_ref7/3, dff_ref3/3, dff_ref4/3, dff_ref5/3, dff_ref1/3, dff_ref2/3, dff2/3, dff3/3, dff8/3, dff9/3, dff1/3, dff13/3, dff14/3, dff11/3, dff10/3, dff15/3, dff16/3, dff12/3, dff6/3, dff7/3, dff5/3, dff4/3
  xor_add23/1 -> xor_add24/2
  xor29/1 -> dbl29/1
  xor_add21/1 -> xor_add22/2
  spike_converter_5/1 -> cvs_in5/1
  xor20/1 -> dbl20/1
  dff_ref13/2 -> xor21/2
  dff_ref9/2 -> xor17/2
  dff_ref12/1 -> dff_ref13/1, xor4/2
  dbl9/1 -> xor_add16/1
  xor28/1 -> dbl28/1
  dff_ref8/1 -> dff_ref9/1, xor32/2
  xor_add11/1 -> xor_add12/2
  dbl24/1 -> xor_add15/2
  dbl6/1 -> xor_add10/1
  dff10/1 -> dff11/1, xor10/1
  spike_converter_1/1 -> cvs_in1/1
  dff_ref3/2 -> xor11/2
  dbl3/1 -> xor_add4/1
  dff2/2 -> xor18/1
  spike_reg/1 -> SPIKE_OUT/1
  dff_ref5/1 -> dff_ref6/1, xor29/2
  dff_ref8/2 -> xor16/2
  dff7/1 -> dff8/1, xor7/1
  xor14/1 -> dbl14/1
  dff_ref16/2 -> dff_ref1/1, xor24/2
  dff4/2 -> xor20/1
  spike_converter_4/1 -> cvs_in4/1
  dff16/2 -> dff1/1, xor32/1
  connections:
  cvs_in4/RConn1 -- rin4/LConn1
  cvs_in1/RConn1 -- rin1/LConn1
  cvs_in3/RConn1 -- rin3/LConn1
  rf/RConn1 -- vout_source/RConn1
  cvs_in5/RConn1 -- rin5/LConn1
  cvs_in2/RConn1 -- rin2/LConn1
  cvs_in5/LConn1 -- vctrl_sense/LConn2 -- vout_source/LConn1 -- gnd/LConn1 -- cvs_in1/LConn1 -- cvs_in3/LConn1 -- cvs_in4/LConn1 -- cvs_in2/LConn1
  vctrl_sense/LConn1 -- rin1/RConn1 -- rin2/RConn1 -- rin3/RConn1 -- rf/LConn1 -- rin5/RConn1 -- rin4/RConn1
